simulink model "Exp3"  (R2020b)
settings: Solver=VariableStepAuto  StartTime=0.0  StopTime=10.0  RelTol=1e-3
libraries: simulink x6, pid_lib x1
settings Model: Creator=geniu  LastModifiedBy=geniu

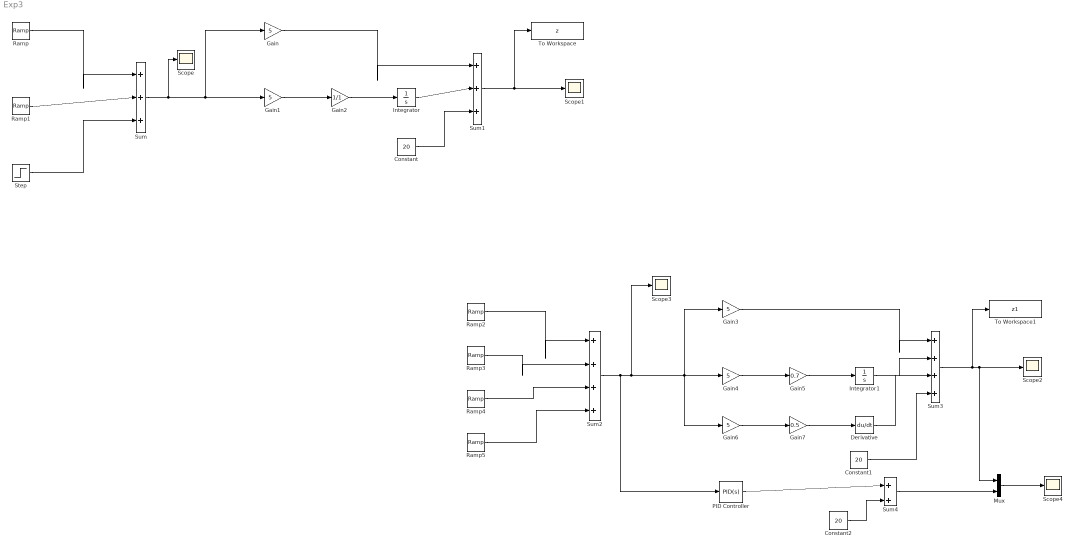
== system Exp3 ==
  Constant : Constant  Value=20
  Constant1 : Constant  Value=20
  Constant2 : Constant  Value=20
  Derivative : Derivative
  Gain{,1,3..4,6} (5 alike) : Gain  Gain=5
  Gain2 : Gain  Gain=1/1
  Gain5 : Gain  Gain=0.7
  Gain7 : Gain  Gain=0.5
  Integrator : Integrator
  Integrator1 : Integrator
  Mux : Mux  Inputs=2
  PID Controller : pid_lib/PID Controller  Controller=PID  Form=Parallel  TimeDomain=Continuous-time  UseExternalTs=off  SampleTime=-1  IntegratorMethod=Forward Euler  FilterMethod=Forward Euler  ControllerParametersSource=internal  P=5  I=3.5  D=2.5  UseFilter=on  N=150  TunerSelectOption=Transfer Function Based (PID Tuner App)  InitialConditionSource=internal  InitialConditionForIntegrator=0  InitialConditionForFilter=0  DifferentiatorICPrevScaledInput=0  ExternalReset=none  TrackingMode=off  Kt=1  LimitOutput=off  SatLimitsSource=internal  UpperSaturationLimit=inf  LowerSaturationLimit=-inf  LinearizeAsGain=on  AntiWindupMode=none  Kb=1  POutMin=[]  POutMax=[]  IOutMin=[]  IOutMax=[]  DOutMin=[]  DOutMax=[]  NOutMin=[]  NOutMax=[]  SumOutMin=[]  SumOutMax=[]  SaturationOutMin=[]  SaturationOutMax=[]  PParamMin=[]  PParamMax=[]  IParamMin=[]  IParamMax=[]  DParamMin=[]  DParamMax=[]  NParamMin=[]  NParamMax=[]  KbParamMin=[]  KbParamMax=[]  KtParamMin=[]  KtParamMax=[]  KbOutMin=[]  KbOutMax=[]  KtOutMin=[]  KtOutMax=[]  IntegratorOutMin=[]  IntegratorOutMax=[]  FilterOutMin=[]  FilterOutMax=[]  SumI1OutMin=[]  SumI1OutMax=[]  SumI2OutMin=[]  SumI2OutMax=[]  SumI3OutMin=[]  SumI3OutMax=[]  SumI4OutMin=[]  SumI4OutMax=[]  SumDOutMin=[]  SumDOutMax=[]  DifferentiatorOutMin=[]  DifferentiatorOutMax=[]  FilterDiffOutCoefMin=[]  FilterDiffOutCoefMax=[]  ReciprocalOutMin=[]  ReciprocalOutMax=[]  SumDenOutMin=[]  SumDenOutMax=[]  SumNumOutMin=[]  SumNumOutMax=[]  DivideOutMin=[]  DivideOutMax=[]  UdiffTsProdOutMin=[]  UdiffTsProdOutMax=[]  NTsProdOutMin=[]  NTsProdOutMax=[]  UintegralTsProdOutMin=[]  UintegralTsProdOutMax=[]  UngainTsProdOutMin=[]  UngainTsProdOutMax=[]  IntegratorContinuousStateAttributes=''  IntegratorStateMustResolveToSignalObject=off  IntegratorRTWStateStorageClass=Auto  FilterContinuousStateAttributes=''  FilterStateMustResolveToSignalObject=off  FilterRTWStateStorageClass=Auto  ParallelPVariant=InternalParameters  IdealPVariant=Disabled  IVariant=InternalParameters  DVariant=InternalParameters  IntegratorVariant=Continuous  SatVariant=Disabled  AWVariant=Passthrough  PCopyVariant=Disabled  TRVariant=Disabled  FdbkBlocksVariant=Forward  IdealPFdbkVariant=Disabled  SatFdbkVariant=Disabled  DerivativeFilterVariant=ContFilter  NVariant=InternalParameters  NCopyVariant=Disabled  FilterICVariant=InternalICsFilter  IntegratorICVariant=InternalICs  ExternalResetVariant=Disabled  TRSumVariant=Passthrough  SumFdbkVariant=Disabled  SumVariant=Sum_PID  TsampFilterVariant=InternalTs  TsampNgainVariant=Passthrough  TsampIntegralVariant=Passthrough  ExternalSaturationOutDataTypeStr=Inherit: Same as second input
  Ramp : simulink/Sources/Ramp  slope=1  start=0  InitialOutput=0
  Ramp1 : simulink/Sources/Ramp  slope=-1  start=1  InitialOutput=0
  Ramp2 : simulink/Sources/Ramp  slope=1  start=0  InitialOutput=0
  Ramp3 : simulink/Sources/Ramp  slope=-1  start=1  InitialOutput=0
  Ramp4 : simulink/Sources/Ramp  slope=-0.5  start=3  InitialOutput=0
  Ramp5 : simulink/Sources/Ramp  slope=0.5  start=5  InitialOutput=0
  Scope{,1..4} (5 alike) : Scope
  Step : Step  Time=3  After=-1  SampleTime=0
  Sum : Sum  Inputs=|+++
  Sum1 : Sum  Inputs=|+++
  Sum2 : Sum  Inputs=|++++
  Sum3 : Sum  Inputs=|++++
  Sum4 : Sum  Inputs=|++
  To Workspace : ToWorkspace  VariableName=z  SampleTime=-1
  To Workspace1 : ToWorkspace  VariableName=z1  SampleTime=-1
  wires:
  Ramp1/1 -> Sum/2
  Ramp/1 -> Sum/1
  Step/1 -> Sum/3
  Sum/1 -> Scope/1, Gain1/1, Gain/1
  Gain2/1 -> Integrator/1
  Gain1/1 -> Gain2/1
  Gain/1 -> Sum1/1
  Sum1/1 -> To Workspace/1, Scope1/1
  Integrator/1 -> Sum1/2
  Constant/1 -> Sum1/3
  Ramp2/1 -> Sum2/1
  Ramp3/1 -> Sum2/2
  Ramp4/1 -> Sum2/3
  Integrator1/1 -> Sum3/2
  Sum3/1 -> Mux/1, Scope2/1, To Workspace1/1
  Gain4/1 -> Gain5/1
  Gain5/1 -> Integrator1/1
  Gain3/1 -> Sum3/1
  Sum2/1 -> Scope3/1, Gain6/1, Gain3/1, Gain4/1, PID Controller/1
  Gain6/1 -> Gain7/1
  Constant1/1 -> Sum3/4
  Gain7/1 -> Derivative/1
  Derivative/1 -> Sum3/3
  Ramp5/1 -> Sum2/4
  Sum4/1 -> Mux/2
  PID Controller/1 -> Sum4/1
  Constant2/1 -> Sum4/2
  Mux/1 -> Scope4/1
